simulink model "Dynamics"  (R2021a)
settings: Solver=VariableStepAuto  StartTime=0.0  StopTime=10.0  RelTol=1e-3
libraries: roblocks x3
settings Model: Creator=root  LastModifiedBy=root

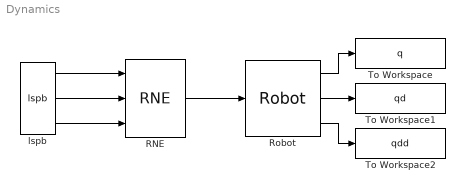
== system Dynamics ==
  RNE : roblocks/Arm/RNE  robot=robot  grav=[0 0 9.81]
  Robot : roblocks/Arm/Robot  robot=robot  q0=[0 0 0 0 0 0]
  To Workspace : ToWorkspace  VariableName=q  SaveFormat=Timeseries  SampleTime=-1
  To Workspace1 : ToWorkspace  VariableName=qd  SaveFormat=Timeseries  SampleTime=-1
  To Workspace2 : ToWorkspace  VariableName=qdd  SaveFormat=Timeseries  SampleTime=-1
  lspb : roblocks/Toolbox/lspb  q0=0  qf=0  tmax=0
  wires:
  RNE/1 -> Robot/1
  lspb/1 -> RNE/1
  lspb/2 -> RNE/2
  lspb/3 -> RNE/3
  Robot/1 -> To Workspace/1
  Robot/2 -> To Workspace1/1
  Robot/3 -> To Workspace2/1
